simulink model "Mode_AOO"  (R2022b)
settings: Solver=FixedStepAuto  StartTime=0.0  StopTime=10.0  FixedStep=1e-3  RelTol=1e-3  EnableMultiTasking=on
undefined symbols (not defined in the file): D10, D11, D12, D2, D4, D5, D7, D8, D9, PTA0, PTA2, PTB23, PTB9, PTC3, PTC4, PTD0, PTD2, PTD3
libraries: frdmk64flib x11
settings Model: ExtModeTrigDuration=5  Creator=sarahalabdulrazzak  LastModifiedBy=sarahalabdulrazzak
settings SolverCC: AlgebraicLoopSolver=TrustRegion
settings OptimizationCC: EnhancedBackFolding=on  PassReuseOutputArgsAs=Individual arguments  ZeroExternalMemoryAtStartup=off  ZeroInternalMemoryAtStartup=off  MaxStackSize=64  OptimizeBlockOrder=speed  DifferentSizesBufferReuse=on  OptimizationCustomize=off  EfficientTunableParamExpr=on
settings DebuggingCC: ParameterTunabilityLossMsg=error  UnconnectedInputMsg=warning  UnconnectedOutputMsg=warning  UnconnectedLineMsg=warning  SFMachineParentedDataDiag=warning
settings HardwareCC: ProdBitPerPointer=32  ProdBitPerSizeT=32  ProdBitPerPtrDiffT=32  ProdLargestAtomicInteger=Long  ProdLargestAtomicFloat=Double  ProdWordSize=32  ProdHWDeviceType=ARM Compatible->ARM Cortex
settings ModelReferenceCC: EnableRefExpFcnMdlSchedulingChecks=on
settings SFSimCC: MATLABDynamicMemAlloc=off
settings RTWCC: Description=Embedded Coder  SystemTargetFile=ert.tlc  HardwareBoard=NXP FRDM-K64F  TLCOptions="-aInlineSetEventsForThisBaseRateFcn=TLC_FALSE -aSuppressMultiTaskScheduler=TLC_FALSE  -aRateBasedStepFcn=0"  TemplateMakefile=ert_default_tmf  Toolchain=GNU Tools for ARM Embedded Processors
settings CodeAppCC: ForceParamTrailComments=on  IgnoreCustomStorageClasses=off  OperatorAnnotations=on  SimulinkDataObjDesc=on  SFDataObjDesc=on  InsertBlockDesc=on

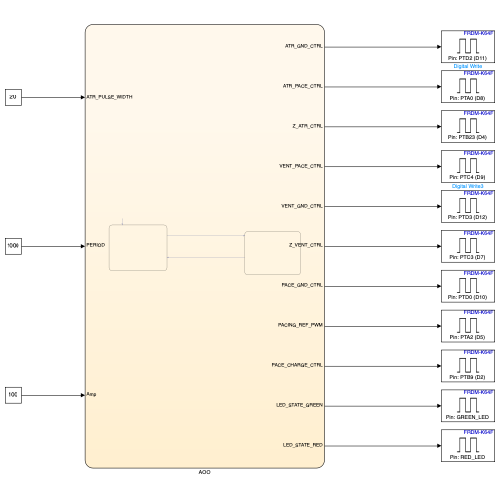
[thumbnail: Simulink's stored preview of the top-level diagram]
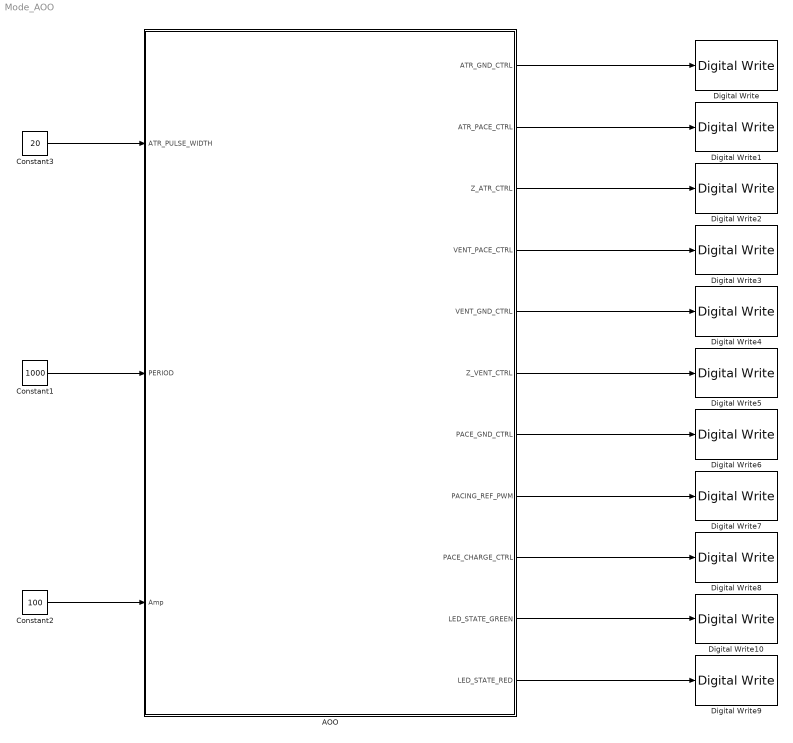
== system Mode_AOO ==
  AOO : Stateflow chart  TreatAsAtomicUnit=on
  Constant1 : Constant  Value=1000
  Constant2 : Constant  Value=100
  Constant3 : Constant  Value=20
  Digital Write : frdmk64flib/Digital Write  Whichpin=PTD2 (D11)
  Digital Write1 : frdmk64flib/Digital Write  Whichpin=PTA0 (D8)
  Digital Write10 : frdmk64flib/Digital Write  Whichpin=GREEN_LED
  Digital Write2 : frdmk64flib/Digital Write  Whichpin=PTB23 (D4)
  Digital Write3 : frdmk64flib/Digital Write  Whichpin=PTC4 (D9)
  Digital Write4 : frdmk64flib/Digital Write  Whichpin=PTD3 (D12)
  Digital Write5 : frdmk64flib/Digital Write  Whichpin=PTC3 (D7)
  Digital Write6 : frdmk64flib/Digital Write  Whichpin=PTD0 (D10)
  Digital Write7 : frdmk64flib/Digital Write  Whichpin=PTA2 (D5)
  Digital Write8 : frdmk64flib/Digital Write  Whichpin=PTB9 (D2)
  Digital Write9 : frdmk64flib/Digital Write  Whichpin=RED_LED
  wires:
  Constant1/1 -> AOO/2(PERIOD)
  Constant2/1 -> AOO/3(Amp)
  Constant3/1 -> AOO/1(ATR_PULSE_WIDTH)
  AOO/1(ATR_GND_CTRL) -> Digital Write/1
  AOO/2(ATR_PACE_CTRL) -> Digital Write1/1
  AOO/3(Z_ATR_CTRL) -> Digital Write2/1
  AOO/4(VENT_PACE_CTRL) -> Digital Write3/1
  AOO/5(VENT_GND_CTRL) -> Digital Write4/1
  AOO/6(Z_VENT_CTRL) -> Digital Write5/1
  AOO/7(PACE_GND_CTRL) -> Digital Write6/1
  AOO/8(PACING_REF_PWM) -> Digital Write7/1
  AOO/9(PACE_CHARGE_CTRL) -> Digital Write8/1
  AOO/11(LED_STATE_RED) -> Digital Write9/1
  AOO/10(LED_STATE_GREEN) -> Digital Write10/1

== stateflow chart Mode_AOO/AOO ==
  state CHARGING
    during:
    %Charge primary capcitor C22
    ATR_PACE_CTRL=LOW
    VENT_PACE_CTRL=LOW
    PACING_REF_PWM = Amp
    PACE_CHARGE_CTRL = HIGH
    %Discharge block capacitor C21
    PACE_GND_CTRL = HIGH
    VENT_PACE_CTRL = LOW
    Z_ATR_CTRL = LOW
    Z_VENT_CTRL = LOW
    ATR_PACE_CTRL = LOW
    ATR_GND_CTRL = HIGH
    VENT_GND_CTRL = LOW
    %Change LED color to verify state
    LED_STATE_RED= true
    LED_STATE_GREEN = false
  state DISCHARGING
    during:
    %Discharge C22 primary capacitor
    %Cahrge C21 block capacitor
    PACE_CHARGE_CTRL = LOW
    PACE_GND_CTRL = HIGH
    ATR_PACE_CTRL = HIGH
    ATR_GND_CTRL = LOW
    Z_ATR_CTRL = LOW
    Z_VENT_CTRL = LOW
    VENT_GND_CTRL = LOW
    VENT_PACE_CTRL  = LOW
    %Change LED color to verify state
    LED_STATE_RED= false
    LED_STATE_GREEN = true
  (default) -> CHARGING
  CHARGING -> DISCHARGING : after(PERIOD - ATR_PULSE_WIDTH,msec)
  DISCHARGING -> CHARGING : after(ATR_PULSE_WIDTH, msec)
  data: ATR_GND_CTRL output; ATR_PACE_CTRL output; Z_ATR_CTRL output; VENT_PACE_CTRL output; VENT_GND_CTRL output; Z_VENT_CTRL output; PACE_GND_CTRL output; PACING_REF_PWM output; PACE_CHARGE_CTRL output; ATR_PULSE_WIDTH input; PERIOD input; HIGH local =true; LOW local =false; LED_STATE_GREEN output; LED_STATE_RED output; Amp input
